simulink model "off_grid_storage"  (R2015b)
settings: Solver=ode45  StartTime=0.0  StopTime=10  RelTol=1e-3
undefined symbols (not defined in the file): Ion, Lithium
libraries: powerlib x49, powerlib_extras x7, electricdrivelib x1
settings Model: Creator=Pouyan  LastModifiedBy=fujitsu
settings DataIOCC: SaveFormat=Array  SignalLoggingSaveFormat=ModelDataLogs
settings OptimizationCC: ExpressionDepthLimit=2147483647
settings DebuggingCC: UnderspecifiedInitializationDetection=Classic  MergeDetectMultiDrivingBlocksExec=none  SolverPrmCheckMsg=warning  FcnCallInpInsideContextMsg=UseLocalSettings  StateNameClashWarn=warning
settings HardwareCC: ProdBitPerPointer=32  ProdLargestAtomicFloat=None  ProdIntDivRoundTo=Undefined  ProdEndianess=Unspecified  ProdWordSize=32  ProdHWDeviceType=32-bit Generic
settings GRTTargetCC: GeneratePreprocessorConditionals=Disable all  CombineOutputUpdateFcns=off  GRTInterface=on
settings ConfigComp: CovModelRefEnable=Off

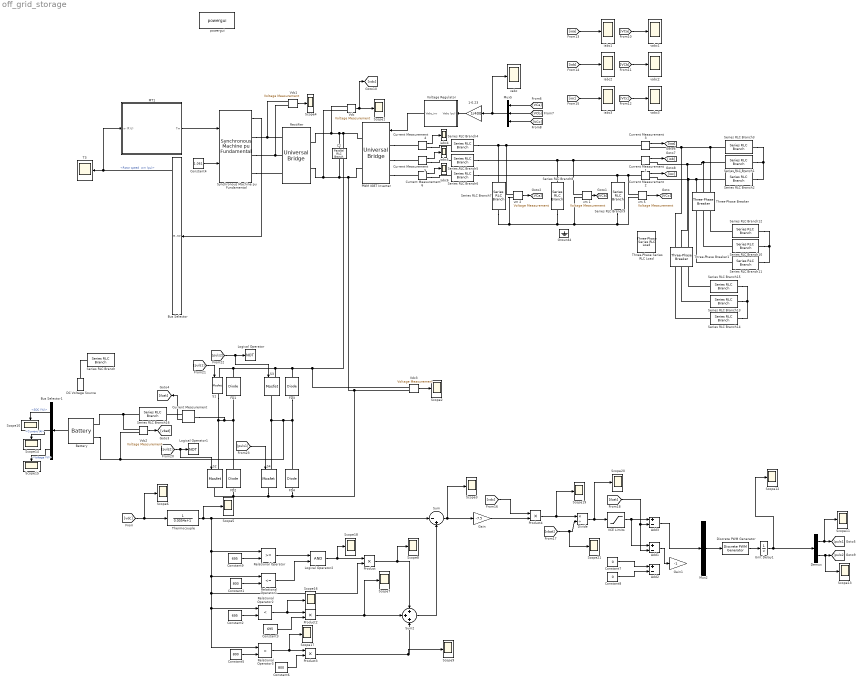
== system off_grid_storage ==
  1-0.23 : Gain  Gain=1/400
  Add1 : Sum  Inputs=+-
  Add2 : Sum  Inputs=+-
  Add3 : Sum  Inputs=+-
  Battery : electricdrivelib/Extra Sources/Battery  BatType=Lithium-Ion  ShowTempParam=off  ThermalPreset=no  NomV=600  NomQ=50  SOC=100  Batt_Tr=10  PresetModel=on  MaxQ=50  FullV=698.3923  Dis_rate=21.7391  R=0.12  Normal_OP=45.2174  expZone="[648.2315      2.456522]"  current=[6.5 13 32.5]  Units=Time  Tci=20  NomT=20  T2=-30  MaxQ2=4.8  FullV2=7.1  Normal_OP2=5.72  expZone2="[6.58  1]"  Rca=0.6  ti=1000
  Bus Selector : BusSelector  OutputSignals="Mechanical.Rotor speed  wm (pu),Stator current. is_a (pu),Stator current. is_b (pu),Stator current. is_c (pu),Mechanical.Electromagnetic torque  Te (pu),Output active power   Peo (pu),Output reactive power  Qeo (pu)"
  Bus Selector1 : BusSelector  OutputSignals=SOC (%),Current (A),Voltage (V)
  C2 : powerlib/Elements/Parallel RLC Branch  LConnTagsString=a  RConnTagsString=__new0  BranchType=C  Resistance=inf  Inductance=inf  SetiL0=off  InitialCurrent=0  Capacitance=5000e-06  Setx0=off  InitialVoltage=0  Measurements=None
  Constant1 : Constant  Value=800
  Constant2 : Constant  Value=695
  Constant3 : Constant  Value=695
  Constant4 : Constant  Value=1.061
  Constant5 : Constant  Value=800
  Constant6 : Constant  Value=800
  Constant7 : Constant  Value=0
  Constant8 : Constant  Value=0
  Constant9 : Constant  Value=695
  Current Measurement{,1..6} (7 alike) : powerlib/Measurements/Current Measurement  PhasorSimulation=off  OutputType=Complex  PSBequivalent=0
  DC Voltage Source : powerlib/Electrical Sources/DC Voltage Source  Amplitude=700  Measurements=None
  Demux : Demux  Outputs=2
  Discrete PWM Generator : powerlib_extras/Discrete  Control Blocks/Discrete PWM Generator  GeneratorMode="1-arm  bridge (2 pulses)"  Fc=2000  Ts=5e-6  Internal=off  mIndex=0.4  Freq=60  Phase=0
  Divide : Product  Inputs=*/
  FD{1..4} (4 alike) : powerlib/Power Electronics/Diode  Ron=0.001  Lon=0  Vf=0.8  IC=0  UseSnubber=off  Rs=500  Cs=250e-9  Measurements=off
  Gain : Gain  Gain=-7.5
  Gain1 : Gain  Gain=-1
  Ground4 : powerlib/Elements/Ground  LConnTagsString=a
  Logical Operator : Logic  Operator=NOT  AllPortsSameDT=off  OutDataTypeStr=boolean
  Logical Operator1 : Logic  Operator=NOT  AllPortsSameDT=off  OutDataTypeStr=boolean
  Logical Operator2 : Logic  AllPortsSameDT=off  OutDataTypeStr=boolean
  MT1 : Subsystem
  Mux2 : Mux  Inputs=1
  Mux5 : Mux  Inputs=3
  PWM IGBT Inverter : powerlib/Power Electronics/Universal Bridge  Arms=3  SnubberResistance=5000  SnubberCapacitance=inf  Device=IGBT / Diodes  Ron=1e-3  Lon=0  ForwardVoltages="[  0.0  0.0  ]"  ForwardVoltage=.8  GTOparameters=[ 1e-6 ,1e-6 ]  IGBTparameters=[ 1e-6 , 2e-6 ]  Measurements=Device currents  Measurements_2=None  converterType=Rectifier
  Product{,2..4} (4 alike) : Product
  Rectifier : powerlib/Power Electronics/Universal Bridge  Arms=3  SnubberResistance=50  SnubberCapacitance=0.1e-6  Device=Diodes  Ron=1e-3  Lon=0  ForwardVoltages="[  0.8  0.8  ]"  ForwardVoltage=.7  GTOparameters=[ 10e-6 , 20e-6 ]  IGBTparameters=[ 1e-6 , 2e-6 ]  Measurements=Device currents  Measurements_2=None  converterType=Rectifier
  Relational Operator : RelationalOperator  OutDataTypeStr=boolean
  Relational Operator1 : RelationalOperator  Operator=<=  OutDataTypeStr=boolean
  Relational Operator2 : RelationalOperator  Operator=<  OutDataTypeStr=boolean
  Relational Operator3 : RelationalOperator  Operator=>  OutDataTypeStr=boolean
  S{1..4} (4 alike) : powerlib/Power Electronics/Mosfet  Ron=0.1  Lon=0  Rd=0.01  Vfd=0  IC=0  Rs=1e5  Cs=inf  Measurements=off
  Scope{1..21} (21 alike) : Scope
  Series RLC Branch : powerlib/Elements/Series RLC Branch  LConnTagsString=__new0  RConnTagsString=__new0  BranchType=R  Resistance=0.0196  Inductance=1e-3  SetiL0=off  InitialCurrent=0  Capacitance=1e-6  Setx0=off  InitialVoltage=0  Measurements=None
  Series RLC Branch1 : powerlib/Elements/Series RLC Branch  LConnTagsString=__new0  RConnTagsString=__new0  BranchType=RL  Resistance=50  Inductance=100e-3  SetiL0=off  InitialCurrent=0  Capacitance=1e-6  Setx0=off  InitialVoltage=0  Measurements=None
  Series RLC Branch10 : powerlib/Elements/Series RLC Branch  LConnTagsString=__new0  RConnTagsString=__new0  BranchType=RL  Resistance=2*50  Inductance=2*100e-3  SetiL0=off  InitialCurrent=0  Capacitance=1e-6  Setx0=off  InitialVoltage=0  Measurements=None
  Series RLC Branch11 : powerlib/Elements/Series RLC Branch  LConnTagsString=__new0  RConnTagsString=__new0  BranchType=RL  Resistance=2*50  Inductance=2*100e-3  SetiL0=off  InitialCurrent=0  Capacitance=1e-6  Setx0=off  InitialVoltage=0  Measurements=None
  Series RLC Branch12 : powerlib/Elements/Series RLC Branch  LConnTagsString=__new0  RConnTagsString=__new0  BranchType=RL  Resistance=2*50  Inductance=2*100e-3  SetiL0=off  InitialCurrent=0  Capacitance=1e-6  Setx0=off  InitialVoltage=0  Measurements=None
  Series RLC Branch13 : powerlib/Elements/Series RLC Branch  LConnTagsString=__new0  RConnTagsString=__new0  BranchType=RL  Resistance=3*50  Inductance=3*100e-3  SetiL0=off  InitialCurrent=0  Capacitance=1e-6  Setx0=off  InitialVoltage=0  Measurements=None
  Series RLC Branch14 : powerlib/Elements/Series RLC Branch  LConnTagsString=__new0  RConnTagsString=__new0  BranchType=RL  Resistance=3*50  Inductance=3*100e-3  SetiL0=off  InitialCurrent=0  Capacitance=1e-6  Setx0=off  InitialVoltage=0  Measurements=None
  Series RLC Branch15 : powerlib/Elements/Series RLC Branch  LConnTagsString=__new0  RConnTagsString=__new0  BranchType=RL  Resistance=3*50  Inductance=3*100e-3  SetiL0=off  InitialCurrent=0  Capacitance=1e-6  Setx0=off  InitialVoltage=0  Measurements=None
  Series RLC Branch16 : powerlib/Elements/Series RLC Branch  LConnTagsString=__new0  RConnTagsString=__new0  BranchType=L  Resistance=0.0196  Inductance=0.004  SetiL0=off  InitialCurrent=0  Capacitance=1e-6  Setx0=off  InitialVoltage=0  Measurements=None
  Series RLC Branch2 : powerlib/Elements/Series RLC Branch  LConnTagsString=__new0  RConnTagsString=__new0  BranchType=RL  Resistance=50  Inductance=100e-3  SetiL0=off  InitialCurrent=0  Capacitance=1e-6  Setx0=off  InitialVoltage=0  Measurements=None
  Series RLC Branch3 : powerlib/Elements/Series RLC Branch  LConnTagsString=__new0  RConnTagsString=__new0  BranchType=RL  Resistance=50  Inductance=100e-3  SetiL0=off  InitialCurrent=0  Capacitance=1e-6  Setx0=off  InitialVoltage=0  Measurements=None
  Series RLC Branch4 : powerlib/Elements/Series RLC Branch  LConnTagsString=__new0  RConnTagsString=__new0  BranchType=L  Resistance=5  Inductance=3e-3  SetiL0=off  InitialCurrent=0  Capacitance=1e-6  Setx0=off  InitialVoltage=0  Measurements=None
  Series RLC Branch5 : powerlib/Elements/Series RLC Branch  LConnTagsString=__new0  RConnTagsString=__new0  BranchType=L  Resistance=5  Inductance=3e-3  SetiL0=off  InitialCurrent=0  Capacitance=1e-6  Setx0=off  InitialVoltage=0  Measurements=None
  Series RLC Branch6 : powerlib/Elements/Series RLC Branch  LConnTagsString=__new0  RConnTagsString=__new0  BranchType=L  Resistance=5  Inductance=3e-3  SetiL0=off  InitialCurrent=0  Capacitance=1e-6  Setx0=off  InitialVoltage=0  Measurements=None
  Series RLC Branch7 : powerlib/Elements/Series RLC Branch  LConnTagsString=__new0  RConnTagsString=__new0  BranchType=C  Resistance=5  Inductance=10e-3  SetiL0=off  InitialCurrent=0  Capacitance=300e-6  Setx0=off  InitialVoltage=0  Measurements=None
  Series RLC Branch8 : powerlib/Elements/Series RLC Branch  LConnTagsString=__new0  RConnTagsString=__new0  BranchType=C  Resistance=5  Inductance=10e-3  SetiL0=off  InitialCurrent=0  Capacitance=300e-6  Setx0=off  InitialVoltage=0  Measurements=None
  Series RLC Branch9 : powerlib/Elements/Series RLC Branch  LConnTagsString=__new0  RConnTagsString=__new0  BranchType=C  Resistance=5  Inductance=10e-3  SetiL0=off  InitialCurrent=0  Capacitance=300e-6  Setx0=off  InitialVoltage=0  Measurements=None
  Sum : Sum  Inputs=|-+
  Sum2 : Sum  Inputs=+++
  Synchronous Machine pu Fundamental : powerlib/Machines/Synchronous Machine pu Fundamental  PresetModel=No  MechanicalLoad=Mechanical power Pm  ShowDetailedParameters=on  RotorType=Salient-pole  Units=per unit fundamental parameters  MeasurementBus=off  NominalParameters="[ 30e3  550 1600]"  Stator="[ 0.2503  0.114  0.6875  0.6875 ]"  Field="[ 1  10e15/(100*pi)]"  Dampers2=[0.0652, 0.5134, 0.0287, 0.2553, 7.765e-3, 0.9167 ]  Dampers1="[ 1.17E-02  0.182  1.97E-02  0.384 ]"  Mechanical=[ 6 0 2]  PolePairs=20  InitialConditions="[ 0  0  0  0  0  0  0  0  1 ]"  SetSaturation=off  Saturation=[0.6404,0.7127,0.8441,0.9214,0.9956,1.082,1.19,1.316,1.457;0.7,0.7698,0.8872,0.9466,0.9969,1.046,1.1,1.151,1.201]  LoadFlowParameters=[1,0,0,0,0]  TsPowergui=0  TsBlock=-1  IterativeModel=Trapezoidal non iterative  BusType=swing  Pref=0  Qref=0  Qmin=-inf  Qmax=inf  PLF=0  QLF=0
  T3 : Scope
  Thermocouple : TransferFcn  Denominator="[0.0054  1]"
  Three-Phase Series RLC Load : powerlib/Elements/Three-Phase Series RLC Load  LConnTagsString=A|B|C  Configuration=Y (grounded)  NominalVoltage=400  Vabc=[1e3 1e3 1e3]  Vabcp=[1e3 1e3 1e3]  NominalFrequency=50  UnbalancedPower=off  ActivePower=20e3  InductivePower=0  CapacitivePower=0  Pabc=[10e3 9e3 11e3]  QLabc=[100 90 110]  QCabc=[100 90 110]  Pabcp=[10e3 9e3 11e3]  QLabcp=[100 90 110]  QCabcp=[100 90 110]  Measurements=None  LoadType=constant Z
  Three-Phase Breaker : powerlib/Elements/Three-Phase Breaker  InitialState=open  SwitchA=on  SwitchB=on  SwitchC=on  SwitchTimes=[4 8]  External=off  BreakerResistance=0.01  SnubberResistance=1e6  SnubberCapacitance=inf  Measurements=None
  Three-Phase Breaker1 : powerlib/Elements/Three-Phase Breaker  InitialState=open  SwitchA=on  SwitchB=on  SwitchC=on  SwitchTimes=[6 8.5]  External=off  BreakerResistance=0.01  SnubberResistance=1e6  SnubberCapacitance=inf  Measurements=None
  Unit Delay1 : UnitDelay  SampleTime=2e-6
  VCE Limits : Saturate  UpperLimit=0.8  LowerLimit=-0.8
  Vdc{,1..3} (4 alike) : powerlib/Measurements/Voltage Measurement  Tag=PoWeRsYsTeMmEaSuReMeNt  PhasorSimulation=off  OutputType=Magnitude  PSBequivalent=0
  Voltage Regulator : Subsystem  mask{kp=0.0001, ki=5}
  iabc{1..6} (6 alike) : Scope
  powergui : powerlib/powergui  SimulationMode=Discrete  SolverType=Tustin  SampleTime=5e-6  frequency=60  SPID=off  DisableSnubberDevices=off  DisableRonSwitches=off  DisableVfSwitches=off  SwTol=0  DisplayEquations=off  Interpol=off  ExternalGateDelay=off  methode=off  Ts=0  FunctionMessages=off  echomessages=off  HookPort=off  EnableUseOfTLC=off  x0status=blocks  frequencyindice=0  Pbase=100e6  ErrMax=0.0001  Iterations=50  UnitsV=kV  UnitsW=MW  buscounter=0  RestoreLinks=warning  ResistiveCurrentMeasurement=off  Frange=[0:2:500]  Ylog=off  Xlog=on  ShowGrid=off  save=off  variable=ZData  structure=Vs  ZoomFFT=on  StartTime=1/60  cycles=1  DisplayStyle=1  fundamental=60  FreqAxis=on  MaxFrequency=10000  frequencyindicesteady=1  RmsSteady=1  display=off
  vabc{,1..3} (4 alike) : Scope
  vm 1 : powerlib/Measurements/Voltage Measurement  PhasorSimulation=off  OutputType=Complex  PSBequivalent=0
  vm 2 : powerlib/Measurements/Voltage Measurement  PhasorSimulation=off  OutputType=Complex  PSBequivalent=0
  vm 5 : powerlib/Measurements/Voltage Measurement  PhasorSimulation=off  OutputType=Complex  PSBequivalent=0
  wires:
  MT1/1(Tm) -> Synchronous Machine pu Fundamental/1
  Synchronous Machine pu Fundamental/1 -> Bus Selector/1
  Constant4/1 -> Synchronous Machine pu Fundamental/2
  Vdc1/1 -> Scope4/1
  Vdc/1 -> [vdc], Scope1/1
  Voltage Regulator/1(Vabc_inv) -> PWM IGBT Inverter/1
  Bus Selector/1 -> MT1/1(w (P.U)), T3/1  "<Rotor speed  wm (pu)>"
  vm 5/1 -> [VCc]
  vm 1/1 -> [VCb]
  vm 2/1 -> [VCa]
  Current Measurement2/1 -> [ioc]
  1-0.23/1 -> Voltage Regulator/1(Vabc (pu))
  [VCa] -> Mux5/1
  [VCb] -> Mux5/2
  [VCc] -> Mux5/3
  Mux5/1 -> vabc/1, 1-0.23/1
  Current Measurement1/1 -> [iob]
  Current Measurement3/1 -> [ioa]
  [VCa] -> vabc1/1
  [VCb] -> vabc2/1
  [VCc] -> vabc3/1
  [ioa] -> iabc1/1
  [iob] -> iabc2/1
  [ioc] -> iabc3/1
  Current Measurement4/1 -> iabc4/1
  Current Measurement5/1 -> iabc5/1
  Current Measurement6/1 -> iabc6/1
  [vdc] -> Scope6/1, Thermocouple/1
  Thermocouple/1 -> Scope5/1, Sum/1, Relational Operator1/1, Product/2, Relational Operator2/1, Relational Operator3/1, Relational Operator/1
  Constant9/1 -> Relational Operator/2
  Product/1 -> Scope8/1, Sum2/1
  Constant1/1 -> Relational Operator1/2
  Relational Operator/1 -> Logical Operator2/1
  Relational Operator1/1 -> Logical Operator2/2
  Logical Operator2/1 -> Scope18/1, Product/1
  Constant2/1 -> Relational Operator2/2
  Relational Operator2/1 -> Scope16/1, Product2/1
  Constant3/1 -> Product2/2
  Product2/1 -> Scope7/1, Sum2/2
  Constant5/1 -> Relational Operator3/2
  Relational Operator3/1 -> Scope17/1, Product3/1
  Constant6/1 -> Product3/2
  Product3/1 -> Scope9/1, Sum2/3
  Sum2/1 -> Sum/2
  Sum/1 -> Scope3/1, Gain/1
  Gain/1 -> Product4/2
  [vdc] -> Product4/1
  Vdc2/1 -> [vbat]
  Product4/1 -> Scope19/1, Divide/1
  [vbat] -> Scope21/1, Divide/2
  Divide/1 -> Scope20/1, VCE Limits/1
  VCE Limits/1 -> Add1/1, Add3/1
  Constant7/1 -> Add2/1
  Constant8/1 -> Add2/2
  Add3/1 -> Mux2/1
  Current Measurement/1 -> [ibat]
  [ibat] -> Add1/2, Add3/2
  Add1/1 -> Gain1/1
  Discrete PWM Generator/1 -> Unit Delay1/1
  Mux2/1 -> Discrete PWM Generator/1
  Unit Delay1/1 -> Scope12/1, Demux/1
  Vdc3/1 -> Scope2/1
  Demux/1 -> Scope11/1, [puls1]
  Demux/2 -> Scope13/1, [puls2]
  [puls2] -> S2/1, Logical Operator1/1
  [puls1] -> S1/1
  [puls1] -> S4/1
  [puls2] -> S3/1, Logical Operator/1
  Battery/1 -> Bus Selector1/1
  Bus Selector1/1 -> Scope10/1  "<SOC (%)>"
  Bus Selector1/2 -> Scope14/1  "<Current (A)>"
  Bus Selector1/3 -> Scope15/1  "<Voltage (V)>"
  connections:
  Synchronous Machine pu Fundamental/RConn1 -- Vdc1/LConn1 -- Rectifier/LConn1
  Synchronous Machine pu Fundamental/RConn2 -- Rectifier/LConn2 -- Vdc1/LConn2
  Synchronous Machine pu Fundamental/RConn3 -- Rectifier/LConn3
  Series RLC Branch3/RConn1 -- Series RLC Branch2/RConn1 -- Series RLC Branch1/RConn1
  vm 2/LConn1 -- Current Measurement3/LConn1 -- Series RLC Branch7/LConn1 -- Series RLC Branch4/RConn1
  Series RLC Branch8/LConn1 -- vm 1/LConn1 -- Current Measurement1/LConn1 -- Series RLC Branch5/RConn1
  vm 5/LConn1 -- Current Measurement2/LConn1 -- Series RLC Branch6/RConn1 -- Series RLC Branch9/LConn1
  vm 5/LConn2 -- Series RLC Branch8/RConn1 -- Series RLC Branch7/RConn1 -- vm 2/LConn2 -- vm 1/LConn2 -- Series RLC Branch9/RConn1
  Series RLC Branch3/LConn1 -- Three-Phase Breaker/LConn3 -- Three-Phase Breaker1/LConn1 -- Current Measurement3/RConn1
  Series RLC Branch1/LConn1 -- Three-Phase Breaker/LConn2 -- Three-Phase Breaker1/LConn2 -- Current Measurement1/RConn1
  Series RLC Branch2/LConn1 -- Three-Phase Breaker/LConn1 -- Three-Phase Breaker1/LConn3 -- Current Measurement2/RConn1
  Current Measurement4/RConn1 -- Series RLC Branch4/LConn1
  PWM IGBT Inverter/LConn1 -- Current Measurement4/LConn1
  Current Measurement5/RConn1 -- Series RLC Branch5/LConn1
  PWM IGBT Inverter/LConn2 -- Current Measurement5/LConn1
  Current Measurement6/RConn1 -- Series RLC Branch6/LConn1
  PWM IGBT Inverter/LConn3 -- Current Measurement6/LConn1
  Vdc2/LConn1 -- Series RLC Branch16/LConn1 -- Battery/LConn1
  S1/RConn1 -- S2/LConn1 -- Current Measurement/LConn1 -- FD1/LConn1 -- FD2/RConn1
  Vdc2/LConn2 -- S3/RConn1 -- S4/LConn1 -- FD3/LConn1 -- FD4/RConn1 -- Battery/LConn2
  Series RLC Branch/LConn1 -- DC Voltage Source/RConn1
  Current Measurement/RConn1 -- Series RLC Branch16/RConn1
  FD4/LConn1 -- Vdc3/LConn2 -- Rectifier/RConn2 -- Vdc/LConn2 -- C2/RConn1 -- PWM IGBT Inverter/RConn2 -- FD2/LConn1 -- S2/RConn1 -- S4/RConn1
  FD1/RConn1 -- S1/LConn1 -- S3/LConn1 -- Vdc3/LConn1 -- PWM IGBT Inverter/RConn1 -- Rectifier/RConn1 -- Vdc/LConn1 -- C2/LConn1 -- FD3/RConn1
  Series RLC Branch12/RConn1 -- Series RLC Branch11/RConn1 -- Series RLC Branch10/RConn1
  Series RLC Branch12/LConn1 -- Three-Phase Breaker/RConn3
  Series RLC Branch10/LConn1 -- Three-Phase Breaker/RConn2
  Series RLC Branch11/LConn1 -- Three-Phase Breaker/RConn1
  Series RLC Branch15/RConn1 -- Series RLC Branch14/RConn1 -- Series RLC Branch13/RConn1
  Series RLC Branch13/LConn1 -- Three-Phase Breaker1/RConn2
  Series RLC Branch15/LConn1 -- Three-Phase Breaker1/RConn3
  Series RLC Branch14/LConn1 -- Three-Phase Breaker1/RConn1

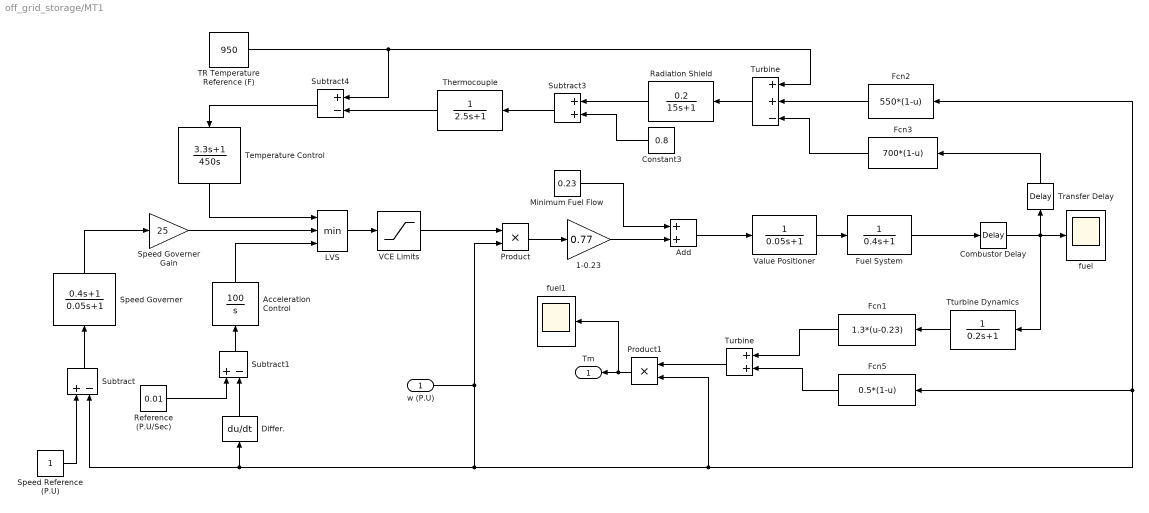
== system off_grid_storage/MT1 ==
  w (P.U) : Inport
  1-0.23 : Gain  Gain=0.77
  Acceleration Control : TransferFcn  Numerator=[0 100]  Denominator=[1 0]
  Add : Sum
  Combustor Delay : TransportDelay  DelayTime=0.01
  Constant3 : Constant  Value=0.8
  Differ. : Derivative
  Fcn1 : Fcn  Expr=1.3*(u-0.23)
  Fcn2 : Fcn  Expr=550*(1-u)
  Fcn3 : Fcn  Expr=700*(1-u)
  Fcn5 : Fcn  Expr=0.5*(1-u)
  Fuel System : TransferFcn  Denominator=[0.4 1]
  LVS : MinMax  Inputs=3
  Minimum Fuel Flow : Constant  Value=0.23
  Product : Product  RndMeth=Zero
  Product1 : Product  RndMeth=Zero
  Radiation Shield : TransferFcn  Numerator=[0.2]  Denominator=[15 1]
  Reference (P.U/Sec) : Constant  Value=0.01
  Speed Governer : TransferFcn  Numerator=[0.4 1]  Denominator=[0.05 1]
  Speed Governer Gain : Gain  Gain=25
  Speed Reference (P.U) : Constant
  Subtract : Sum  Inputs=+-
  Subtract1 : Sum  Inputs=+-
  Subtract3 : Sum
  Subtract4 : Sum  Inputs=+-
  TR Temperature Reference (F) : Constant  Value=950
  Temperature Control : TransferFcn  Numerator=[3.3 1]  Denominator=[450 0]
  Thermocouple : TransferFcn  Denominator=[2.5 1]
  Transfer Delay : TransportDelay  DelayTime=0.04
  Tturbine Dynamics : TransferFcn  Denominator=[0.2 1]
  Turbine : Sum  Inputs=++-
  "Turbine " : Sum
  VCE Limits : Saturate  UpperLimit=1.5  LowerLimit=-0.1
  Value Positioner : TransferFcn  Denominator=[0.05 1]
  fuel : Scope
  fuel1 : Scope
  Tm : Outport
  wires:
  "Turbine "/1 -> Product1/1
  Product1/1 -> fuel1/1, Tm/1
  Fcn5/1 -> "Turbine "/2
  Fcn1/1 -> "Turbine "/1
  Tturbine Dynamics/1 -> Fcn1/1
  w (P.U)/1 -> Fcn2/1, Fcn5/1, Product1/2, Differ./1, Subtract/2, Product/2
  Speed Governer/1 -> Speed Governer Gain/1
  Temperature Control/1 -> LVS/1
  Subtract4/1 -> Temperature Control/1
  TR Temperature Reference (F)/1 -> Subtract4/1, Turbine/1
  Thermocouple/1 -> Subtract4/2
  Subtract3/1 -> Thermocouple/1
  Turbine/1 -> Radiation Shield/1
  Constant3/1 -> Subtract3/2
  Radiation Shield/1 -> Subtract3/1
  Fcn2/1 -> Turbine/2
  Fcn3/1 -> Turbine/3
  Transfer Delay/1 -> Fcn3/1
  LVS/1 -> VCE Limits/1
  Acceleration Control/1 -> LVS/3
  Subtract1/1 -> Acceleration Control/1
  Reference (P.U/Sec)/1 -> Subtract1/1
  Differ./1 -> Subtract1/2
  Speed Governer Gain/1 -> LVS/2
  Combustor Delay/1 -> Tturbine Dynamics/1, fuel/1, Transfer Delay/1
  Fuel System/1 -> Combustor Delay/1
  Value Positioner/1 -> Fuel System/1
  Add/1 -> Value Positioner/1
  Minimum Fuel Flow/1 -> Add/1
  1-0.23/1 -> Add/2
  Product/1 -> 1-0.23/1
  VCE Limits/1 -> Product/1
  Subtract/1 -> Speed Governer/1
  Speed Reference (P.U)/1 -> Subtract/1

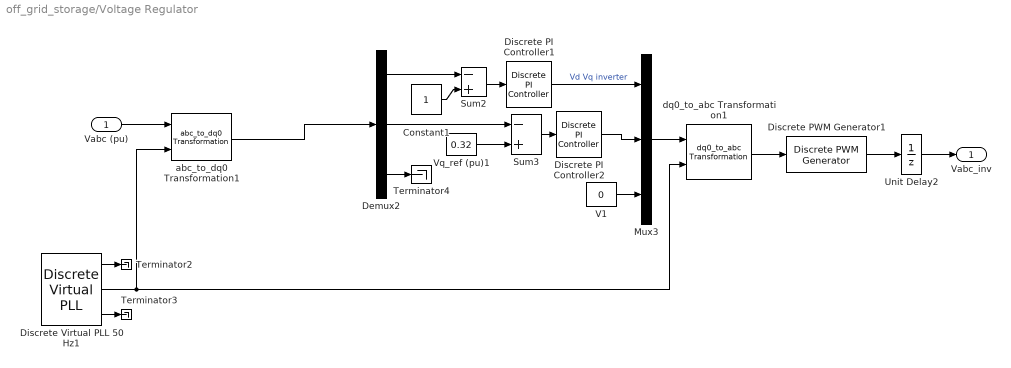
== system off_grid_storage/Voltage Regulator ==
  Vabc (pu) : Inport
  Constant1 : Constant
  Demux2 : Demux  Outputs=3
  Discrete PI Controller1 : powerlib_extras/Discrete  Control Blocks/Discrete PI Controller  Kp=kp  Ki=ki  Par_Limits=[1 -1]  Init=0  Ts=5e-6
  Discrete PI Controller2 : powerlib_extras/Discrete  Control Blocks/Discrete PI Controller  Kp=kp  Ki=ki  Par_Limits=[1 -1]  Init=0  Ts=5e-6
  Discrete PWM Generator1 : powerlib_extras/Discrete  Control Blocks/Discrete PWM Generator  GeneratorMode="3-arm  bridge (6 pulses)"  Fc=2000  Ts=5e-6  Internal=off  mIndex=0.4  Freq=60  Phase=0
  Discrete Virtual PLL 50 Hz1 : powerlib_extras/Discrete  Control Blocks/Discrete Virtual PLL  Freq=50  Phase=0  Ts=5e-6
  Mux3 : Mux  Inputs=3
  Sum2 : Sum  Inputs=-+  SaturateOnIntegerOverflow=on  InputSameDT=on  OutDataTypeStr=Inherit: Same as first input
  Sum3 : Sum  Inputs=-+  SaturateOnIntegerOverflow=on  InputSameDT=on  OutDataTypeStr=Inherit: Same as first input
  Terminator2 : Terminator
  Terminator3 : Terminator
  Terminator4 : Terminator
  Unit Delay2 : UnitDelay  SampleTime=5e-6
  V1 : Constant  Value=0
  Vq_ref (pu)1 : Constant  Value=0.32
  abc_to_dq0 Transformation1 : powerlib_extras/Measurements/abc_to_dq0 Transformation
  dq0_to_abc Transformation1 : powerlib_extras/Measurements/dq0_to_abc Transformation
  Vabc_inv : Outport
  wires:
  Demux2/1 -> Sum2/1
  Sum2/1 -> Discrete PI Controller1/1
  Mux3/1 -> dq0_to_abc Transformation1/1
  Discrete Virtual PLL 50 Hz1/2 -> abc_to_dq0 Transformation1/2, dq0_to_abc Transformation1/2
  Discrete Virtual PLL 50 Hz1/1 -> Terminator2/1
  Discrete Virtual PLL 50 Hz1/3 -> Terminator3/1
  Discrete PWM Generator1/1 -> Unit Delay2/1
  abc_to_dq0 Transformation1/1 -> Demux2/1
  Demux2/3 -> Terminator4/1
  Constant1/1 -> Sum2/2
  Demux2/2 -> Sum3/1
  Vq_ref (pu)1/1 -> Sum3/2
  Sum3/1 -> Discrete PI Controller2/1
  Discrete PI Controller1/1 -> Mux3/1  "Vd Vq inverter"
  Discrete PI Controller2/1 -> Mux3/2
  V1/1 -> Mux3/3
  Unit Delay2/1 -> Vabc_inv/1
  Vabc (pu)/1 -> abc_to_dq0 Transformation1/1
  dq0_to_abc Transformation1/1 -> Discrete PWM Generator1/1
